simulink model "SF106A_MotRplCoggCfg"  (R2013b)
settings: Solver=FixedStepDiscrete  SolverMode=SingleTasking  StartTime=0.0  StopTime=1  FixedStep=0.002  RelTol=1e-3
undefined symbols (not defined in the file): ARCHGLBPRM_2PI_ULS_F32, ARCHGLBPRM_FLOATZEROTHD_ULS_F32, ARCHGLBPRM_HALFSQRT3_ULS_F32, COGGORDER1_CNT_U16, COGGORDER2_CNT_U16, COGGORDER3_CNT_U16, magnitude, MotCtrlPrmEstimnMotBackEmfConNom, MotRplCoggCfgMotAgTiDly, MotRplCoggCfgMotCurrDaxRplBilnrSeln, MotRplCoggCfgMotCurrQaxRpl, MotRplCoggCfgMotTqRplOrder1X, MotRplCoggCfgMotTqRplOrder1Y, MotRplCoggCfgMotTqRplOrder2X, MotRplCoggCfgMotTqRplOrder2Y, MotRplCoggCfgMotTqRplOrder3X, MotRplCoggCfgMotTqRplOrder3Y, MotRplCoggCmdHrmncOrder1Elec, MotRplCoggCmdHrmncOrder2Elec, MotRplCoggCmdHrmncOrder3Elec, NvmGetErrSts1, ONEOVER2_ULS_F32, SysGlbPrmMotPoleCnt, THREEOVER8_ULS_F32
libraries: NxtrLim x20, FixdToFloat x12, FloatToFixd x6, BilnrIntrpnCmnX x6, BilnrIntrpnCmnXDyn x6, NxtrMath x6, NxtrAbslt x5, NxtrNvM x3, simulink x2, NxtrSign x2
(part 3 of 3)

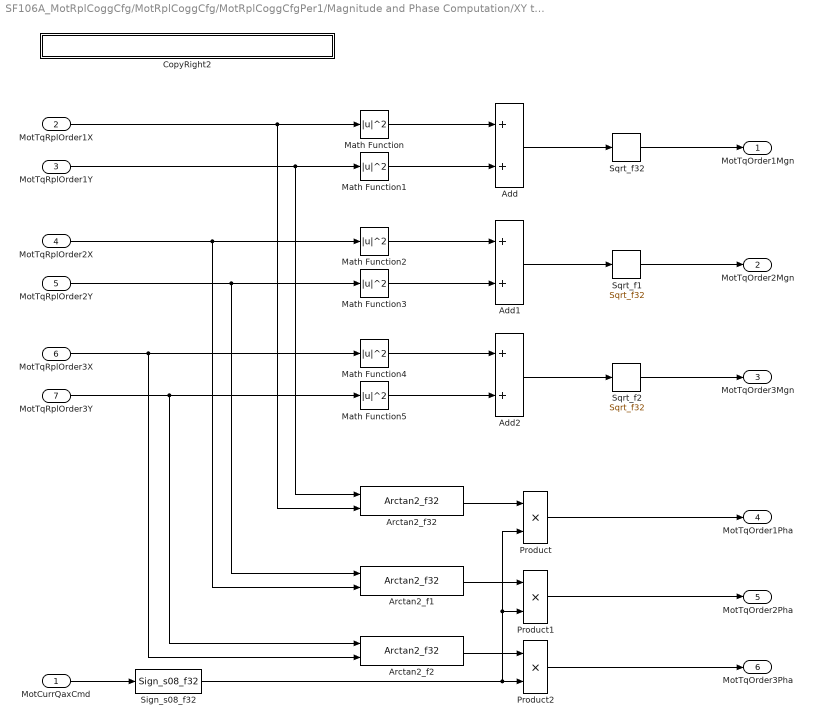
== system SF106A_MotRplCoggCfg/MotRplCoggCfg/MotRplCoggCfgPer1/Magnitude and Phase Computation/XY to Magnitude and Phase ==
  MotCurrQaxCmd : Inport
  MotTqRplOrder1X : Inport  Port=2
  MotTqRplOrder1Y : Inport  Port=3
  MotTqRplOrder2X : Inport  Port=4
  MotTqRplOrder2Y : Inport  Port=5
  MotTqRplOrder3X : Inport  Port=6
  MotTqRplOrder3Y : Inport  Port=7
  Add : Sum  RequirementInfo="{'linktype_rmi_doors' '0000bb45 (/E-STEER Core/SubSystem Specifications/Application Functions/SF99/SF106A Cogging and Ripple Configuration)' '#SF106A_61' 'true' 'REQ:  SF106A_61' '' } %GIDa_e125a99c_4a2f_459a_9981_14e8024e171e"
  Add1 : Sum  RequirementInfo="{'linktype_rmi_doors' '0000bb45 (/E-STEER Core/SubSystem Specifications/Application Functions/SF99/SF106A Cogging and Ripple Configuration)' '#SF106A_61' 'true' 'REQ:  SF106A_61' '' } %GIDa_16906b26_eee0_4222_8977_aa153b29a4e6"
  Add2 : Sum  RequirementInfo="{'linktype_rmi_doors' '0000bb45 (/E-STEER Core/SubSystem Specifications/Application Functions/SF99/SF106A Cogging and Ripple Configuration)' '#SF106A_61' 'true' 'REQ:  SF106A_61' '' } %GIDa_f2bba23d_5da9_4e25_be78_966662a480fc"
  Arctan2_f1 : NxtrMath/Arctan2_f32  RequirementInfo="{'linktype_rmi_doors' '0000bb45 (/E-STEER Core/SubSystem Specifications/Application Functions/SF99/SF106A Cogging and Ripple Configuration)' '#SF106A_61' 'true' 'REQ:  SF106A_61' '' } %GIDa_cc3245e9_b693_4e50_8aea_4d9cc7cbf071"  SFunctionSpec=single y1 = Arctan2_f32(single u1, single u2)
      settings: AttributesFormatString=%<MaskType>
  Arctan2_f2 : NxtrMath/Arctan2_f32  RequirementInfo="{'linktype_rmi_doors' '0000bb45 (/E-STEER Core/SubSystem Specifications/Application Functions/SF99/SF106A Cogging and Ripple Configuration)' '#SF106A_61' 'true' 'REQ:  SF106A_61' '' } %GIDa_2189325a_b245_4b5e_9a63_534dccbdb28e"  SFunctionSpec=single y1 = Arctan2_f32(single u1, single u2)
      settings: AttributesFormatString=%<MaskType>
  Arctan2_f32 : NxtrMath/Arctan2_f32  RequirementInfo="{'linktype_rmi_doors' '0000bb45 (/E-STEER Core/SubSystem Specifications/Application Functions/SF99/SF106A Cogging and Ripple Configuration)' '#SF106A_61' 'true' 'REQ:  SF106A_61' '' } %GIDa_7ad43da0_66d8_42f2_936c_146a54904ef1"  SFunctionSpec=single y1 = Arctan2_f32(single u1, single u2)
      settings: AttributesFormatString=%<MaskType>
  CopyRight2 : Subsystem  Description=|  mask(Copyright Information){none=on}
      | Copyright info block.                                               
      |                                                                     
      | Place copyright information at the top of every subsystem in design.
      mask prompts: none "No parameters"
      mask help: Place copyright information at the top of every subsystem in design.
      mask Display:
      | NxtrConf = 'Nexteer Confidential';
      | 
      | sys = bdroot; %handle for the current model ("system")
      | first = get_param(sys,'Created');
      | if(isempty(first))
      |     first = datestr(now,'yyyy');
      | else
      |     first = first(end-3:end);  %year is last four digits
      | end
      | 
      | last = get_param(sys,'LastModifiedDate');
      | if isempty(last)
      |     last = datestr(now,'yyyy');
      | else
      |     last = last(end-3:end);
      | end
      | 
      | if strcmp(first,last)
      |     fprintf('%s -- Copyright %s Nexteer',NxtrConf,first)
      | else
      |     fprintf('%s -- %s%s- %s Nexteer',NxtrConf,char(169),first,last)
      | end
  Math Function : Math  RequirementInfo="{'linktype_rmi_doors' '0000bb45 (/E-STEER Core/SubSystem Specifications/Application Functions/SF99/SF106A Cogging and Ripple Configuration)' '#SF106A_61' 'true' 'REQ:  SF106A_61' '' } %GIDa_d8cc266b_04e4_485b_ae87_42220da5313a"  Operator=magnitude^2  SaturateOnIntegerOverflow=on
  Math Function1 : Math  RequirementInfo="{'linktype_rmi_doors' '0000bb45 (/E-STEER Core/SubSystem Specifications/Application Functions/SF99/SF106A Cogging and Ripple Configuration)' '#SF106A_61' 'true' 'REQ:  SF106A_61' '' } %GIDa_99b757f3_b84e_41d8_85ec_0f2d477d9e0c"  Operator=magnitude^2  SaturateOnIntegerOverflow=on
  Math Function2 : Math  RequirementInfo="{'linktype_rmi_doors' '0000bb45 (/E-STEER Core/SubSystem Specifications/Application Functions/SF99/SF106A Cogging and Ripple Configuration)' '#SF106A_61' 'true' 'REQ:  SF106A_61' '' } %GIDa_d527198d_19fb_41d2_9f46_025eabacc3a0"  Operator=magnitude^2  SaturateOnIntegerOverflow=on
  Math Function3 : Math  RequirementInfo="{'linktype_rmi_doors' '0000bb45 (/E-STEER Core/SubSystem Specifications/Application Functions/SF99/SF106A Cogging and Ripple Configuration)' '#SF106A_61' 'true' 'REQ:  SF106A_61' '' } %GIDa_a2580a3c_c18e_4b9f_afca_32fe8dbf9a20"  Operator=magnitude^2  SaturateOnIntegerOverflow=on
  Math Function4 : Math  RequirementInfo="{'linktype_rmi_doors' '0000bb45 (/E-STEER Core/SubSystem Specifications/Application Functions/SF99/SF106A Cogging and Ripple Configuration)' '#SF106A_61' 'true' 'REQ:  SF106A_61' '' } %GIDa_a199d0d4_c905_44ea_9143_52d6147e94a8"  Operator=magnitude^2  SaturateOnIntegerOverflow=on
  Math Function5 : Math  RequirementInfo="{'linktype_rmi_doors' '0000bb45 (/E-STEER Core/SubSystem Specifications/Application Functions/SF99/SF106A Cogging and Ripple Configuration)' '#SF106A_61' 'true' 'REQ:  SF106A_61' '' } %GIDa_506a2bc7_f63d_4fb6_8e52_caa68cc33753"  Operator=magnitude^2  SaturateOnIntegerOverflow=on
  Product : Product
  Product1 : Product
  Product2 : Product
  Sign_s08_f32 : NxtrSign/Sign_s08_f32  RequirementInfo="{'linktype_rmi_doors' '0000bb45 (/E-STEER Core/SubSystem Specifications/Application Functions/SF99/SF106A Cogging and Ripple Configuration)' '#SF106A_61' 'true' 'REQ:  SF106A_61' '' } %GIDa_77a62122_400e_4984_a30a_ec753c60c126"  SFunctionSpec=int8 y1 = Sign_s08_f32(single u1)
  Sqrt_f1 : NxtrMath/Sqrt_f32  RequirementInfo="{'linktype_rmi_doors' '0000bb45 (/E-STEER Core/SubSystem Specifications/Application Functions/SF99/SF106A Cogging and Ripple Configuration)' '#SF106A_61' 'true' 'REQ:  SF106A_61' '' } %GIDa_fd8bed59_24cc_4d74_927b_0c2c5c223437"  SFunctionSpec=single y1 = Sqrt_f32(single u1)  ShowSpec=on
      settings: AttributesFormatString=%<MaskType>
  Sqrt_f2 : NxtrMath/Sqrt_f32  RequirementInfo="{'linktype_rmi_doors' '0000bb45 (/E-STEER Core/SubSystem Specifications/Application Functions/SF99/SF106A Cogging and Ripple Configuration)' '#SF106A_61' 'true' 'REQ:  SF106A_61' '' } %GIDa_912b3a84_5d7d_4607_a083_8be65564d9aa"  SFunctionSpec=single y1 = Sqrt_f32(single u1)  ShowSpec=on
      settings: AttributesFormatString=%<MaskType>
  Sqrt_f32 : NxtrMath/Sqrt_f32  RequirementInfo="{'linktype_rmi_doors' '0000bb45 (/E-STEER Core/SubSystem Specifications/Application Functions/SF99/SF106A Cogging and Ripple Configuration)' '#SF106A_61' 'true' 'REQ:  SF106A_61' '' } %GIDa_9efcafb4_d419_487c_951d_011ca062ed91"  SFunctionSpec=single y1 = Sqrt_f32(single u1)  ShowSpec=on
      settings: AttributesFormatString=%<MaskType>
  MotTqOrder1Mgn : Outport
  MotTqOrder2Mgn : Outport  Port=2
  MotTqOrder3Mgn : Outport  Port=3
  MotTqOrder1Pha : Outport  Port=4
  MotTqOrder2Pha : Outport  Port=5
  MotTqOrder3Pha : Outport  Port=6
  wires:
  MotTqRplOrder1X/1 -> Arctan2_f32/2, Math Function/1
  MotTqRplOrder1Y/1 -> Arctan2_f32/1, Math Function1/1
  MotTqRplOrder3Y/1 -> Arctan2_f2/1, Math Function5/1
  MotTqRplOrder3X/1 -> Arctan2_f2/2, Math Function4/1
  MotTqRplOrder2Y/1 -> Arctan2_f1/1, Math Function3/1
  MotTqRplOrder2X/1 -> Arctan2_f1/2, Math Function2/1
  Math Function/1 -> Add/1
  Math Function1/1 -> Add/2
  Math Function2/1 -> Add1/1
  Math Function3/1 -> Add1/2
  Math Function4/1 -> Add2/1
  Math Function5/1 -> Add2/2
  Add/1 -> Sqrt_f32/1
  Add1/1 -> Sqrt_f1/1
  Add2/1 -> Sqrt_f2/1
  MotCurrQaxCmd/1 -> Sign_s08_f32/1
  Sqrt_f32/1 -> MotTqOrder1Mgn/1
  Product2/1 -> MotTqOrder3Pha/1
  Product1/1 -> MotTqOrder2Pha/1
  Sqrt_f2/1 -> MotTqOrder3Mgn/1
  Sqrt_f1/1 -> MotTqOrder2Mgn/1
  Product/1 -> MotTqOrder1Pha/1
  Arctan2_f32/1 -> Product/1
  Sign_s08_f32/1 -> Product2/2, Product/2, Product1/2
  Arctan2_f1/1 -> Product1/1
  Arctan2_f2/1 -> Product2/1

== system SF106A_MotRplCoggCfg/MotRplCoggCfg/MotRplCoggCfgPer1/MotCurrToMotTqGain Calc/CopyRight2 ==

== system SF106A_MotRplCoggCfg/MotRplCoggCfg/MotRplCoggCfgPer1/MotCurrToMotTqGain Calc/Output Directly ==
  In1 : Inport
  Action Port : ActionPort  ActionType=else
  CopyRight2 : Subsystem  Description=|  mask(Copyright Information){none=on}
      | Copyright info block.                                               
      |                                                                     
      | Place copyright information at the top of every subsystem in design.
      mask prompts: none "No parameters"
      mask help: Place copyright information at the top of every subsystem in design.
      mask Display:
      | NxtrConf = 'Nexteer Confidential';
      | 
      | sys = bdroot; %handle for the current model ("system")
      | first = get_param(sys,'Created');
      | if(isempty(first))
      |     first = datestr(now,'yyyy');
      | else
      |     first = first(end-3:end);  %year is last four digits
      | end
      | 
      | last = get_param(sys,'LastModifiedDate');
      | if isempty(last)
      |     last = datestr(now,'yyyy');
      | else
      |     last = last(end-3:end);
      | end
      | 
      | if strcmp(first,last)
      |     fprintf('%s -- Copyright %s Nexteer',NxtrConf,first)
      | else
      |     fprintf('%s -- %s%s- %s Nexteer',NxtrConf,char(169),first,last)
      | end
  Out1 : Outport
  wires:
  In1/1 -> Out1/1

== system SF106A_MotRplCoggCfg/MotRplCoggCfg/MotRplCoggCfgPer1/MotCurrToMotTqGain Calc/Set to Default ==
  MotBackEmfConEstimd : Inport
  Action Port : ActionPort  ActionType=then
  Constant4 : Constant  Value=ARCHGLBPRM_HALFSQRT3_ULS_F32
  CopyRight2 : Subsystem  Description=|  mask(Copyright Information){none=on}
      | Copyright info block.                                               
      |                                                                     
      | Place copyright information at the top of every subsystem in design.
      mask prompts: none "No parameters"
      mask help: Place copyright information at the top of every subsystem in design.
      mask Display:
      | NxtrConf = 'Nexteer Confidential';
      | 
      | sys = bdroot; %handle for the current model ("system")
      | first = get_param(sys,'Created');
      | if(isempty(first))
      |     first = datestr(now,'yyyy');
      | else
      |     first = first(end-3:end);  %year is last four digits
      | end
      | 
      | last = get_param(sys,'LastModifiedDate');
      | if isempty(last)
      |     last = datestr(now,'yyyy');
      | else
      |     last = last(end-3:end);
      | end
      | 
      | if strcmp(first,last)
      |     fprintf('%s -- Copyright %s Nexteer',NxtrConf,first)
      | else
      |     fprintf('%s -- %s%s- %s Nexteer',NxtrConf,char(169),first,last)
      | end
  Product1 : Product
  Out1 : Outport
  wires:
  MotBackEmfConEstimd/1 -> Product1/1
  Product1/1 -> Out1/1
  Constant4/1 -> Product1/2

== system SF106A_MotRplCoggCfg/MotRplCoggCfg/MotRplCoggCfgPer1/Position Delay/CopyRight2 ==

== system SF106A_MotRplCoggCfg/MotRplCoggCfg/MotRplCoggCfgPer1/Magnitude and Phase Computation/Current Regulator Bandwidth Compensation/CopyRight2 ==

== system SF106A_MotRplCoggCfg/MotRplCoggCfg/MotRplCoggCfgPer1/Magnitude and Phase Computation/Current Regulator Bandwidth Compensation/Order 1  Response ==
  MotTqCmdScad : Inport
  MotVelOrder1Hrmnc : Inport  Port=2
  BilnrIntrpnWithRound_u16_u16CmnXu16MplY : BilnrIntrpnCmnX/BilnrIntrpnWithRound_u16_u16CmnXu16MplY  XTbl=MotRplCoggCfgMotTqCmdCurrRgltrBwCmpX  MplYTbl=MotRplCoggCfgMotTqCmdCurrRgltrBwCmpMgnY  BilnrSelnTbl=MotRplCoggCfgMotVelBilnrSeln
      settings: AttributesFormatString=Bilnr ( u16CmnX , u16MplY )
  BilnrIntrpnWithRound_u16_u16CmnXu16MplY1 : BilnrIntrpnCmnX/BilnrIntrpnWithRound_u16_u16CmnXu16MplY  XTbl=MotRplCoggCfgMotTqCmdCurrRgltrBwCmpX  MplYTbl=MotRplCoggCfgMotTqCmdCurrRgltrBwCmpPhaY  BilnrSelnTbl=MotRplCoggCfgMotVelBilnrSeln
      settings: AttributesFormatString=Bilnr ( u16CmnX , u16MplY )
  CopyRight2 : Subsystem  Description=|  mask(Copyright Information){none=on}
      | Copyright info block.                                               
      |                                                                     
      | Place copyright information at the top of every subsystem in design.
      mask prompts: none "No parameters"
      mask help: Place copyright information at the top of every subsystem in design.
      mask Display:
      | NxtrConf = 'Nexteer Confidential';
      | 
      | sys = bdroot; %handle for the current model ("system")
      | first = get_param(sys,'Created');
      | if(isempty(first))
      |     first = datestr(now,'yyyy');
      | else
      |     first = first(end-3:end);  %year is last four digits
      | end
      | 
      | last = get_param(sys,'LastModifiedDate');
      | if isempty(last)
      |     last = datestr(now,'yyyy');
      | else
      |     last = last(end-3:end);
      | end
      | 
      | if strcmp(first,last)
      |     fprintf('%s -- Copyright %s Nexteer',NxtrConf,first)
      | else
      |     fprintf('%s -- %s%s- %s Nexteer',NxtrConf,char(169),first,last)
      | end
  Order1MgnCmp : Outport
  Order1PhaCmp : Outport  Port=2
  wires:
  MotTqCmdScad/1 -> BilnrIntrpnWithRound_u16_u16CmnXu16MplY1/1, BilnrIntrpnWithRound_u16_u16CmnXu16MplY/1
  MotVelOrder1Hrmnc/1 -> BilnrIntrpnWithRound_u16_u16CmnXu16MplY1/2, BilnrIntrpnWithRound_u16_u16CmnXu16MplY/2
  BilnrIntrpnWithRound_u16_u16CmnXu16MplY/1 -> Order1MgnCmp/1
  BilnrIntrpnWithRound_u16_u16CmnXu16MplY1/1 -> Order1PhaCmp/1

== system SF106A_MotRplCoggCfg/MotRplCoggCfg/MotRplCoggCfgPer1/Magnitude and Phase Computation/Current Regulator Bandwidth Compensation/Order 2 Response ==
  MotTqCmdScad : Inport
  MotVelOrder2Hrmnc : Inport  Port=2
  BilnrIntrpnWithRound_u16_u16CmnXu16MplY : BilnrIntrpnCmnX/BilnrIntrpnWithRound_u16_u16CmnXu16MplY  XTbl=MotRplCoggCfgMotTqCmdCurrRgltrBwCmpX  MplYTbl=MotRplCoggCfgMotTqCmdCurrRgltrBwCmpMgnY  BilnrSelnTbl=MotRplCoggCfgMotVelBilnrSeln
      settings: AttributesFormatString=Bilnr ( u16CmnX , u16MplY )
  BilnrIntrpnWithRound_u16_u16CmnXu16MplY1 : BilnrIntrpnCmnX/BilnrIntrpnWithRound_u16_u16CmnXu16MplY  XTbl=MotRplCoggCfgMotTqCmdCurrRgltrBwCmpX  MplYTbl=MotRplCoggCfgMotTqCmdCurrRgltrBwCmpPhaY  BilnrSelnTbl=MotRplCoggCfgMotVelBilnrSeln
      settings: AttributesFormatString=Bilnr ( u16CmnX , u16MplY )
  CopyRight2 : Subsystem  Description=|  mask(Copyright Information){none=on}
      | Copyright info block.                                               
      |                                                                     
      | Place copyright information at the top of every subsystem in design.
      mask prompts: none "No parameters"
      mask help: Place copyright information at the top of every subsystem in design.
      mask Display:
      | NxtrConf = 'Nexteer Confidential';
      | 
      | sys = bdroot; %handle for the current model ("system")
      | first = get_param(sys,'Created');
      | if(isempty(first))
      |     first = datestr(now,'yyyy');
      | else
      |     first = first(end-3:end);  %year is last four digits
      | end
      | 
      | last = get_param(sys,'LastModifiedDate');
      | if isempty(last)
      |     last = datestr(now,'yyyy');
      | else
      |     last = last(end-3:end);
      | end
      | 
      | if strcmp(first,last)
      |     fprintf('%s -- Copyright %s Nexteer',NxtrConf,first)
      | else
      |     fprintf('%s -- %s%s- %s Nexteer',NxtrConf,char(169),first,last)
      | end
  Order2MgnCmp : Outport
  Order2PhaCmp : Outport  Port=2
  wires:
  BilnrIntrpnWithRound_u16_u16CmnXu16MplY1/1 -> Order2PhaCmp/1
  BilnrIntrpnWithRound_u16_u16CmnXu16MplY/1 -> Order2MgnCmp/1
  MotVelOrder2Hrmnc/1 -> BilnrIntrpnWithRound_u16_u16CmnXu16MplY/2, BilnrIntrpnWithRound_u16_u16CmnXu16MplY1/2
  MotTqCmdScad/1 -> BilnrIntrpnWithRound_u16_u16CmnXu16MplY/1, BilnrIntrpnWithRound_u16_u16CmnXu16MplY1/1

== system SF106A_MotRplCoggCfg/MotRplCoggCfg/MotRplCoggCfgPer1/Magnitude and Phase Computation/Current Regulator Bandwidth Compensation/Order 3 Response ==
  MotTqCmdScad : Inport
  MotVelOrder3Hrmnc : Inport  Port=2
  BilnrIntrpnWithRound_u16_u16CmnXu16MplY : BilnrIntrpnCmnX/BilnrIntrpnWithRound_u16_u16CmnXu16MplY  XTbl=MotRplCoggCfgMotTqCmdCurrRgltrBwCmpX  MplYTbl=MotRplCoggCfgMotTqCmdCurrRgltrBwCmpMgnY  BilnrSelnTbl=MotRplCoggCfgMotVelBilnrSeln
      settings: AttributesFormatString=Bilnr ( u16CmnX , u16MplY )
  BilnrIntrpnWithRound_u16_u16CmnXu16MplY1 : BilnrIntrpnCmnX/BilnrIntrpnWithRound_u16_u16CmnXu16MplY  XTbl=MotRplCoggCfgMotTqCmdCurrRgltrBwCmpX  MplYTbl=MotRplCoggCfgMotTqCmdCurrRgltrBwCmpPhaY  BilnrSelnTbl=MotRplCoggCfgMotVelBilnrSeln
      settings: AttributesFormatString=Bilnr ( u16CmnX , u16MplY )
  CopyRight2 : Subsystem  Description=|  mask(Copyright Information){none=on}
      | Copyright info block.                                               
      |                                                                     
      | Place copyright information at the top of every subsystem in design.
      mask prompts: none "No parameters"
      mask help: Place copyright information at the top of every subsystem in design.
      mask Display:
      | NxtrConf = 'Nexteer Confidential';
      | 
      | sys = bdroot; %handle for the current model ("system")
      | first = get_param(sys,'Created');
      | if(isempty(first))
      |     first = datestr(now,'yyyy');
      | else
      |     first = first(end-3:end);  %year is last four digits
      | end
      | 
      | last = get_param(sys,'LastModifiedDate');
      | if isempty(last)
      |     last = datestr(now,'yyyy');
      | else
      |     last = last(end-3:end);
      | end
      | 
      | if strcmp(first,last)
      |     fprintf('%s -- Copyright %s Nexteer',NxtrConf,first)
      | else
      |     fprintf('%s -- %s%s- %s Nexteer',NxtrConf,char(169),first,last)
      | end
  Order3MgnCmp : Outport
  Order3PhaCmp : Outport  Port=2
  wires:
  MotTqCmdScad/1 -> BilnrIntrpnWithRound_u16_u16CmnXu16MplY/1, BilnrIntrpnWithRound_u16_u16CmnXu16MplY1/1
  MotVelOrder3Hrmnc/1 -> BilnrIntrpnWithRound_u16_u16CmnXu16MplY1/2, BilnrIntrpnWithRound_u16_u16CmnXu16MplY/2
  BilnrIntrpnWithRound_u16_u16CmnXu16MplY/1 -> Order3MgnCmp/1
  BilnrIntrpnWithRound_u16_u16CmnXu16MplY1/1 -> Order3PhaCmp/1

== system SF106A_MotRplCoggCfg/MotRplCoggCfg/MotRplCoggCfgPer1/Magnitude and Phase Computation/Torque Ripple Base/CopyRight2 ==

== system SF106A_MotRplCoggCfg/MotRplCoggCfg/MotRplCoggCfgPer1/Magnitude and Phase Computation/Wrap Order1 Phase/CopyRight2 ==

== system SF106A_MotRplCoggCfg/MotRplCoggCfg/MotRplCoggCfgPer1/Magnitude and Phase Computation/Wrap Order1 Phase/If Action Subsystem1 ==
  Action Port : ActionPort  ActionType=then
  Constant9 : Constant  Value=ARCHGLBPRM_2PI_ULS_F32
  CopyRight2 : Subsystem  Description=|  mask(Copyright Information){none=on}
      | Copyright info block.                                               
      |                                                                     
      | Place copyright information at the top of every subsystem in design.
      mask prompts: none "No parameters"
      mask help: Place copyright information at the top of every subsystem in design.
      mask Display:
      | NxtrConf = 'Nexteer Confidential';
      | 
      | sys = bdroot; %handle for the current model ("system")
      | first = get_param(sys,'Created');
      | if(isempty(first))
      |     first = datestr(now,'yyyy');
      | else
      |     first = first(end-3:end);  %year is last four digits
      | end
      | 
      | last = get_param(sys,'LastModifiedDate');
      | if isempty(last)
      |     last = datestr(now,'yyyy');
      | else
      |     last = last(end-3:end);
      | end
      | 
      | if strcmp(first,last)
      |     fprintf('%s -- Copyright %s Nexteer',NxtrConf,first)
      | else
      |     fprintf('%s -- %s%s- %s Nexteer',NxtrConf,char(169),first,last)
      | end
  Out1 : Outport
  wires:
  Constant9/1 -> Out1/1

== system SF106A_MotRplCoggCfg/MotRplCoggCfg/MotRplCoggCfgPer1/Magnitude and Phase Computation/Wrap Order1 Phase/If Action Subsystem2 ==
  Action Port : ActionPort  ActionType=elseif
  Constant9 : Constant  Value=ARCHGLBPRM_2PI_ULS_F32
  CopyRight2 : Subsystem  Description=|  mask(Copyright Information){none=on}
      | Copyright info block.                                               
      |                                                                     
      | Place copyright information at the top of every subsystem in design.
      mask prompts: none "No parameters"
      mask help: Place copyright information at the top of every subsystem in design.
      mask Display:
      | NxtrConf = 'Nexteer Confidential';
      | 
      | sys = bdroot; %handle for the current model ("system")
      | first = get_param(sys,'Created');
      | if(isempty(first))
      |     first = datestr(now,'yyyy');
      | else
      |     first = first(end-3:end);  %year is last four digits
      | end
      | 
      | last = get_param(sys,'LastModifiedDate');
      | if isempty(last)
      |     last = datestr(now,'yyyy');
      | else
      |     last = last(end-3:end);
      | end
      | 
      | if strcmp(first,last)
      |     fprintf('%s -- Copyright %s Nexteer',NxtrConf,first)
      | else
      |     fprintf('%s -- %s%s- %s Nexteer',NxtrConf,char(169),first,last)
      | end
  Unary Minus : UnaryMinus
  Out1 : Outport
  wires:
  Constant9/1 -> Unary Minus/1
  Unary Minus/1 -> Out1/1

== system SF106A_MotRplCoggCfg/MotRplCoggCfg/MotRplCoggCfgPer1/Magnitude and Phase Computation/Wrap Order1 Phase/If Action Subsystem5 ==
  Action Port : ActionPort  ActionType=else
  Constant1 : Constant  Value=0  OutDataTypeStr=single
      settings: AttributesFormatString=%<OutDataTypeStr>
  CopyRight2 : Subsystem  Description=|  mask(Copyright Information){none=on}
      | Copyright info block.                                               
      |                                                                     
      | Place copyright information at the top of every subsystem in design.
      mask prompts: none "No parameters"
      mask help: Place copyright information at the top of every subsystem in design.
      mask Display:
      | NxtrConf = 'Nexteer Confidential';
      | 
      | sys = bdroot; %handle for the current model ("system")
      | first = get_param(sys,'Created');
      | if(isempty(first))
      |     first = datestr(now,'yyyy');
      | else
      |     first = first(end-3:end);  %year is last four digits
      | end
      | 
      | last = get_param(sys,'LastModifiedDate');
      | if isempty(last)
      |     last = datestr(now,'yyyy');
      | else
      |     last = last(end-3:end);
      | end
      | 
      | if strcmp(first,last)
      |     fprintf('%s -- Copyright %s Nexteer',NxtrConf,first)
      | else
      |     fprintf('%s -- %s%s- %s Nexteer',NxtrConf,char(169),first,last)
      | end
  Out1 : Outport
  wires:
  Constant1/1 -> Out1/1

== system SF106A_MotRplCoggCfg/MotRplCoggCfg/MotRplCoggCfgPer1/Magnitude and Phase Computation/Wrap Order2 Phase/CopyRight2 ==

== system SF106A_MotRplCoggCfg/MotRplCoggCfg/MotRplCoggCfgPer1/Magnitude and Phase Computation/Wrap Order2 Phase/If Action Subsystem1 ==
  Action Port : ActionPort  ActionType=then
  Constant9 : Constant  Value=ARCHGLBPRM_2PI_ULS_F32
  CopyRight2 : Subsystem  Description=|  mask(Copyright Information){none=on}
      | Copyright info block.                                               
      |                                                                     
      | Place copyright information at the top of every subsystem in design.
      mask prompts: none "No parameters"
      mask help: Place copyright information at the top of every subsystem in design.
      mask Display:
      | NxtrConf = 'Nexteer Confidential';
      | 
      | sys = bdroot; %handle for the current model ("system")
      | first = get_param(sys,'Created');
      | if(isempty(first))
      |     first = datestr(now,'yyyy');
      | else
      |     first = first(end-3:end);  %year is last four digits
      | end
      | 
      | last = get_param(sys,'LastModifiedDate');
      | if isempty(last)
      |     last = datestr(now,'yyyy');
      | else
      |     last = last(end-3:end);
      | end
      | 
      | if strcmp(first,last)
      |     fprintf('%s -- Copyright %s Nexteer',NxtrConf,first)
      | else
      |     fprintf('%s -- %s%s- %s Nexteer',NxtrConf,char(169),first,last)
      | end
  Out1 : Outport
  wires:
  Constant9/1 -> Out1/1

== system SF106A_MotRplCoggCfg/MotRplCoggCfg/MotRplCoggCfgPer1/Magnitude and Phase Computation/Wrap Order2 Phase/If Action Subsystem2 ==
  Action Port : ActionPort  ActionType=elseif
  Constant9 : Constant  Value=ARCHGLBPRM_2PI_ULS_F32
  CopyRight2 : Subsystem  Description=|  mask(Copyright Information){none=on}
      | Copyright info block.                                               
      |                                                                     
      | Place copyright information at the top of every subsystem in design.
      mask prompts: none "No parameters"
      mask help: Place copyright information at the top of every subsystem in design.
      mask Display:
      | NxtrConf = 'Nexteer Confidential';
      | 
      | sys = bdroot; %handle for the current model ("system")
      | first = get_param(sys,'Created');
      | if(isempty(first))
      |     first = datestr(now,'yyyy');
      | else
      |     first = first(end-3:end);  %year is last four digits
      | end
      | 
      | last = get_param(sys,'LastModifiedDate');
      | if isempty(last)
      |     last = datestr(now,'yyyy');
      | else
      |     last = last(end-3:end);
      | end
      | 
      | if strcmp(first,last)
      |     fprintf('%s -- Copyright %s Nexteer',NxtrConf,first)
      | else
      |     fprintf('%s -- %s%s- %s Nexteer',NxtrConf,char(169),first,last)
      | end
  Unary Minus : UnaryMinus
  Out1 : Outport
  wires:
  Unary Minus/1 -> Out1/1
  Constant9/1 -> Unary Minus/1

== system SF106A_MotRplCoggCfg/MotRplCoggCfg/MotRplCoggCfgPer1/Magnitude and Phase Computation/Wrap Order2 Phase/If Action Subsystem5 ==
  Action Port : ActionPort  ActionType=else
  Constant1 : Constant  Value=0  OutDataTypeStr=single
      settings: AttributesFormatString=%<OutDataTypeStr>
  CopyRight2 : Subsystem  Description=|  mask(Copyright Information){none=on}
      | Copyright info block.                                               
      |                                                                     
      | Place copyright information at the top of every subsystem in design.
      mask prompts: none "No parameters"
      mask help: Place copyright information at the top of every subsystem in design.
      mask Display:
      | NxtrConf = 'Nexteer Confidential';
      | 
      | sys = bdroot; %handle for the current model ("system")
      | first = get_param(sys,'Created');
      | if(isempty(first))
      |     first = datestr(now,'yyyy');
      | else
      |     first = first(end-3:end);  %year is last four digits
      | end
      | 
      | last = get_param(sys,'LastModifiedDate');
      | if isempty(last)
      |     last = datestr(now,'yyyy');
      | else
      |     last = last(end-3:end);
      | end
      | 
      | if strcmp(first,last)
      |     fprintf('%s -- Copyright %s Nexteer',NxtrConf,first)
      | else
      |     fprintf('%s -- %s%s- %s Nexteer',NxtrConf,char(169),first,last)
      | end
  Out1 : Outport
  wires:
  Constant1/1 -> Out1/1

== system SF106A_MotRplCoggCfg/MotRplCoggCfg/MotRplCoggCfgPer1/Magnitude and Phase Computation/Wrap Order3 Phase/CopyRight2 ==

== system SF106A_MotRplCoggCfg/MotRplCoggCfg/MotRplCoggCfgPer1/Magnitude and Phase Computation/Wrap Order3 Phase/If Action Subsystem1 ==
  Action Port : ActionPort  ActionType=then
  Constant9 : Constant  Value=ARCHGLBPRM_2PI_ULS_F32
  CopyRight2 : Subsystem  Description=|  mask(Copyright Information){none=on}
      | Copyright info block.                                               
      |                                                                     
      | Place copyright information at the top of every subsystem in design.
      mask prompts: none "No parameters"
      mask help: Place copyright information at the top of every subsystem in design.
      mask Display:
      | NxtrConf = 'Nexteer Confidential';
      | 
      | sys = bdroot; %handle for the current model ("system")
      | first = get_param(sys,'Created');
      | if(isempty(first))
      |     first = datestr(now,'yyyy');
      | else
      |     first = first(end-3:end);  %year is last four digits
      | end
      | 
      | last = get_param(sys,'LastModifiedDate');
      | if isempty(last)
      |     last = datestr(now,'yyyy');
      | else
      |     last = last(end-3:end);
      | end
      | 
      | if strcmp(first,last)
      |     fprintf('%s -- Copyright %s Nexteer',NxtrConf,first)
      | else
      |     fprintf('%s -- %s%s- %s Nexteer',NxtrConf,char(169),first,last)
      | end
  Out1 : Outport
  wires:
  Constant9/1 -> Out1/1

== system SF106A_MotRplCoggCfg/MotRplCoggCfg/MotRplCoggCfgPer1/Magnitude and Phase Computation/Wrap Order3 Phase/If Action Subsystem2 ==
  Action Port : ActionPort  ActionType=elseif
  Constant9 : Constant  Value=ARCHGLBPRM_2PI_ULS_F32
  CopyRight2 : Subsystem  Description=|  mask(Copyright Information){none=on}
      | Copyright info block.                                               
      |                                                                     
      | Place copyright information at the top of every subsystem in design.
      mask prompts: none "No parameters"
      mask help: Place copyright information at the top of every subsystem in design.
      mask Display:
      | NxtrConf = 'Nexteer Confidential';
      | 
      | sys = bdroot; %handle for the current model ("system")
      | first = get_param(sys,'Created');
      | if(isempty(first))
      |     first = datestr(now,'yyyy');
      | else
      |     first = first(end-3:end);  %year is last four digits
      | end
      | 
      | last = get_param(sys,'LastModifiedDate');
      | if isempty(last)
      |     last = datestr(now,'yyyy');
      | else
      |     last = last(end-3:end);
      | end
      | 
      | if strcmp(first,last)
      |     fprintf('%s -- Copyright %s Nexteer',NxtrConf,first)
      | else
      |     fprintf('%s -- %s%s- %s Nexteer',NxtrConf,char(169),first,last)
      | end
  Unary Minus : UnaryMinus
  Out1 : Outport
  wires:
  Constant9/1 -> Unary Minus/1
  Unary Minus/1 -> Out1/1

== system SF106A_MotRplCoggCfg/MotRplCoggCfg/MotRplCoggCfgPer1/Magnitude and Phase Computation/Wrap Order3 Phase/If Action Subsystem5 ==
  Action Port : ActionPort  ActionType=else
  Constant1 : Constant  Value=0  OutDataTypeStr=single
      settings: AttributesFormatString=%<OutDataTypeStr>
  CopyRight2 : Subsystem  Description=|  mask(Copyright Information){none=on}
      | Copyright info block.                                               
      |                                                                     
      | Place copyright information at the top of every subsystem in design.
      mask prompts: none "No parameters"
      mask help: Place copyright information at the top of every subsystem in design.
      mask Display:
      | NxtrConf = 'Nexteer Confidential';
      | 
      | sys = bdroot; %handle for the current model ("system")
      | first = get_param(sys,'Created');
      | if(isempty(first))
      |     first = datestr(now,'yyyy');
      | else
      |     first = first(end-3:end);  %year is last four digits
      | end
      | 
      | last = get_param(sys,'LastModifiedDate');
      | if isempty(last)
      |     last = datestr(now,'yyyy');
      | else
      |     last = last(end-3:end);
      | end
      | 
      | if strcmp(first,last)
      |     fprintf('%s -- Copyright %s Nexteer',NxtrConf,first)
      | else
      |     fprintf('%s -- %s%s- %s Nexteer',NxtrConf,char(169),first,last)
      | end
  Out1 : Outport
  wires:
  Constant1/1 -> Out1/1

== system SF106A_MotRplCoggCfg/MotRplCoggCfg/MotRplCoggCfgPer1/Magnitude and Phase Computation/XY to Magnitude and Phase/CopyRight2 ==

== system SF106A_MotRplCoggCfg/MotRplCoggCfg/MotRplCoggCfgPer1/MotCurrToMotTqGain Calc/Output Directly/CopyRight2 ==

== system SF106A_MotRplCoggCfg/MotRplCoggCfg/MotRplCoggCfgPer1/MotCurrToMotTqGain Calc/Set to Default/CopyRight2 ==

== system SF106A_MotRplCoggCfg/MotRplCoggCfg/MotRplCoggCfgPer1/Magnitude and Phase Computation/Current Regulator Bandwidth Compensation/Order 1  Response/CopyRight2 ==

== system SF106A_MotRplCoggCfg/MotRplCoggCfg/MotRplCoggCfgPer1/Magnitude and Phase Computation/Current Regulator Bandwidth Compensation/Order 2 Response/CopyRight2 ==

== system SF106A_MotRplCoggCfg/MotRplCoggCfg/MotRplCoggCfgPer1/Magnitude and Phase Computation/Current Regulator Bandwidth Compensation/Order 3 Response/CopyRight2 ==

== system SF106A_MotRplCoggCfg/MotRplCoggCfg/MotRplCoggCfgPer1/Magnitude and Phase Computation/Wrap Order1 Phase/If Action Subsystem1/CopyRight2 ==

== system SF106A_MotRplCoggCfg/MotRplCoggCfg/MotRplCoggCfgPer1/Magnitude and Phase Computation/Wrap Order1 Phase/If Action Subsystem2/CopyRight2 ==

== system SF106A_MotRplCoggCfg/MotRplCoggCfg/MotRplCoggCfgPer1/Magnitude and Phase Computation/Wrap Order1 Phase/If Action Subsystem5/CopyRight2 ==

== system SF106A_MotRplCoggCfg/MotRplCoggCfg/MotRplCoggCfgPer1/Magnitude and Phase Computation/Wrap Order2 Phase/If Action Subsystem1/CopyRight2 ==

== system SF106A_MotRplCoggCfg/MotRplCoggCfg/MotRplCoggCfgPer1/Magnitude and Phase Computation/Wrap Order2 Phase/If Action Subsystem2/CopyRight2 ==

== system SF106A_MotRplCoggCfg/MotRplCoggCfg/MotRplCoggCfgPer1/Magnitude and Phase Computation/Wrap Order2 Phase/If Action Subsystem5/CopyRight2 ==

== system SF106A_MotRplCoggCfg/MotRplCoggCfg/MotRplCoggCfgPer1/Magnitude and Phase Computation/Wrap Order3 Phase/If Action Subsystem1/CopyRight2 ==

== system SF106A_MotRplCoggCfg/MotRplCoggCfg/MotRplCoggCfgPer1/Magnitude and Phase Computation/Wrap Order3 Phase/If Action Subsystem2/CopyRight2 ==

== system SF106A_MotRplCoggCfg/MotRplCoggCfg/MotRplCoggCfgPer1/Magnitude and Phase Computation/Wrap Order3 Phase/If Action Subsystem5/CopyRight2 ==
